simulink model "restapi_master_task"  (Simulink 3.00)
undefined symbols (not defined in the file): application, json
libraries: stringlib x3, mathlib x2, speclib x2, genlib x1, logiclib x1

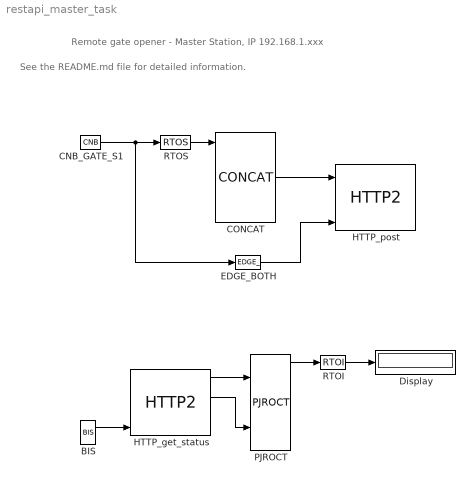
== system restapi_master_task ==
  note: See the README.md file for detailed information.
  note: Remote gate opener - Master Station, IP 192.168.1.xxx
  BIS : genlib/BIS  Y0=on  t1=0.1  t2=5  t3=0  t4=4  t5=5  t6=6  t7=7  t8=8  RPT=on
  CNB_GATE_S1 : mathlib/CNB  YCN=off
  CONCAT : stringlib/CONCAT  ptrn="{ \"v\": %1}"  nmax=0
  Display : Display
      settings: Format=Best fit
  EDGE_BOTH : logiclib/EDGE_  iedge=3: Both edges
  HTTP_get_status : speclib/HTTP2  url=http://192.168.1.101:8008/api/tasks/restapi_slave_task/Gate:OPENED  method=1: GET  user=admin  VERIFY=off  postmime=application/json  acceptmime=application/json  timeout=5  BLOCKING=off  nmax=0  postmax=256  datamax=1024
  HTTP_post : speclib/HTTP2  url=http://192.168.1.101:8008/api/tasks/restapi_slave_task/CNB_GATE:YCN  method=2: POST  user=admin  VERIFY=off  postmime=application/json  acceptmime=application/json  timeout=5  BLOCKING=off  nmax=0  postmax=256  datamax=1024
  PJROCT : stringlib/PJROCT  name1=v  nmax=0  yerr=0
  RTOI : mathlib/RTOI
  RTOS : stringlib/RTOS  prec=0  mode=1: best fit
  wires:
  BIS/1 -> HTTP_get_status/4
  CNB_GATE_S1/1 -> EDGE_BOTH/1, RTOS/1
  CONCAT/1 -> HTTP_post/1
  EDGE_BOTH/1 -> HTTP_post/4
  HTTP_get_status/1 -> PJROCT/1
  HTTP_get_status/3 -> PJROCT/2
  PJROCT/1 -> RTOI/1
  RTOI/1 -> Display/1
  RTOS/1 -> CONCAT/1
